simulink model "Controlador_PI"  (R2023a)
settings: Solver=ode1  StartTime=0.0  StopTime=10.0  FixedStep=0.01  RelTol=1e-3
settings Model: Creator=Nacho Andrade  LastModifiedBy=Nacho Andrade

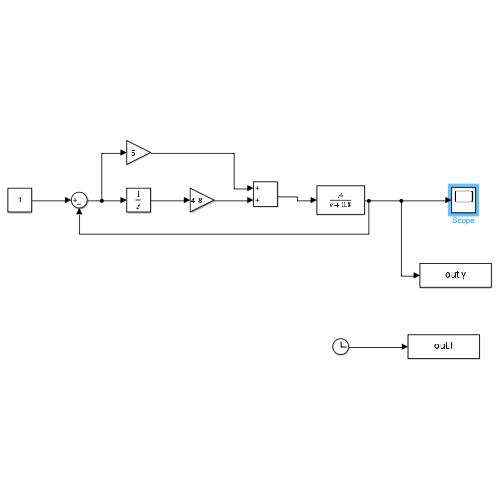
[thumbnail: Simulink's stored preview of the top-level diagram]
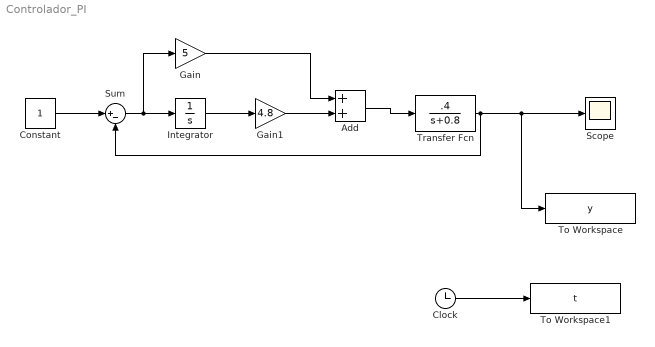
== system Controlador_PI ==
  Add : Sum
  Clock : Clock
  Constant : Constant
  Gain : Gain  Gain=5
  Gain1 : Gain  Gain=4.8
  Integrator : Integrator
  Scope : Scope
  Sum : Sum  Inputs=|+-
  To Workspace : ToWorkspace  VariableName=y  SampleTime=-1
  To Workspace1 : ToWorkspace  VariableName=t  SampleTime=-1
  Transfer Fcn : TransferFcn  Numerator=[.4]  Denominator=[1 0.8]
  wires:
  Constant/1 -> Sum/1
  Integrator/1 -> Gain1/1
  Sum/1 -> Gain/1, Integrator/1
  Transfer Fcn/1 -> Sum/2, To Workspace/1, Scope/1
  Gain1/1 -> Add/2
  Add/1 -> Transfer Fcn/1
  Gain/1 -> Add/1
  Clock/1 -> To Workspace1/1
